simulink model "RC_withsignal_testing"  (R2023a)
settings: Solver=VariableStepAuto  StartTime=0.0  StopTime=10.0  FixedStep=0.001  MaxStep=0.001  RelTol=1e-3
libraries: simulink x1
settings Model: Creator=alaam  LastModifiedBy=alaam

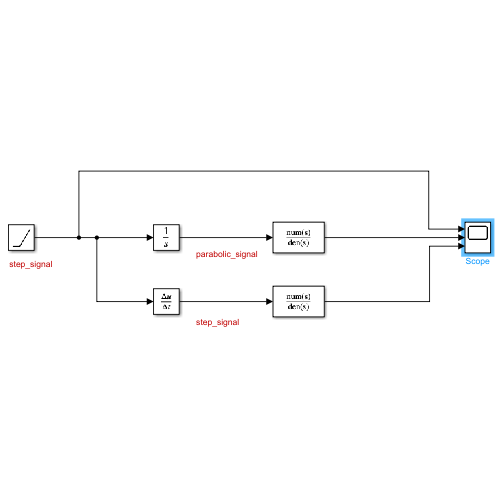
[thumbnail: Simulink's stored preview of the top-level diagram]
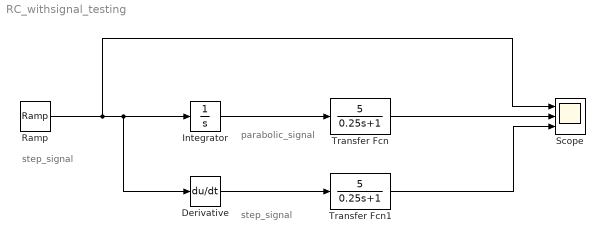
== system RC_withsignal_testing ==
  note: step_signal
  note: parabolic_signal
  note: step_signal
  Derivative : Derivative
  Integrator : Integrator
  Ramp : simulink/Sources/Ramp  slope=2  start=0  InitialOutput=0
  Scope : Scope  NumInputPorts=3
  Transfer Fcn : TransferFcn  Numerator=[0 5]  Denominator=[0.25 1]
  Transfer Fcn1 : TransferFcn  Numerator=[0 5]  Denominator=[0.25 1]
  wires:
  Ramp/1 -> Scope/1, Derivative/1, Integrator/1
  Integrator/1 -> Transfer Fcn/1
  Derivative/1 -> Transfer Fcn1/1
  Transfer Fcn/1 -> Scope/2
  Transfer Fcn1/1 -> Scope/3
